simulink model "a3_P1"  (R2023b)
settings: Solver=VariableStepAuto  StartTime=0.0  StopTime=0.2  MaxStep=0.001  RelTol=1e-3
settings Model: Creator=amandeepbehera  LastModifiedBy=amandeepbehera

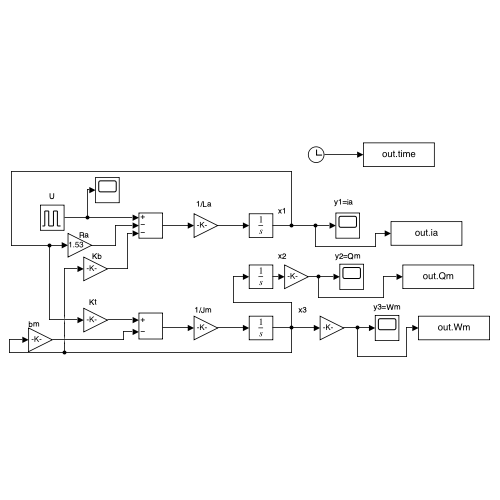
[thumbnail: Simulink's stored preview of the top-level diagram]
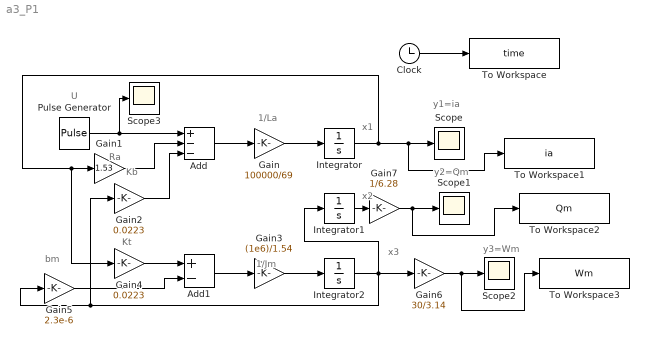
== system a3_P1 ==
  note: y3=Wm
  note: y2=Qm
  note: y1=ia
  note: x3
  note: bm
  note: Kt
  note: 1/Jm
  note: x2
  note: x1
  note: Kb
  note: Ra
  note: U
  note: 1/La
  Add : Sum  Inputs=+--
  Add1 : Sum  Inputs=+-
  Clock : Clock
  Gain : Gain  Gain=100000/69
  Gain1 : Gain  Gain=1.53
  Gain2 : Gain  Gain=0.0223
  Gain3 : Gain  Gain=(1e6)/1.54
  Gain4 : Gain  Gain=0.0223
  Gain5 : Gain  Gain=2.3e-6
  Gain6 : Gain  Gain=30/3.14
  Gain7 : Gain  Gain=1/6.28
  Integrator : Integrator
  Integrator1 : Integrator
  Integrator2 : Integrator
  Pulse Generator : DiscretePulseGenerator  PulseType=Time based  Amplitude=10  Period=.2  PulseWidth=50
  Scope{,1..3} (4 alike) : Scope
  To Workspace : ToWorkspace  VariableName=time  SampleTime=-1
  To Workspace1 : ToWorkspace  VariableName=ia  SampleTime=-1
  To Workspace2 : ToWorkspace  VariableName=Qm  SampleTime=-1
  To Workspace3 : ToWorkspace  VariableName=Wm  SampleTime=-1
  wires:
  Add/1 -> Gain/1
  Gain/1 -> Integrator/1
  Integrator/1 -> To Workspace1/1, Scope/1, Gain4/1, Gain1/1
  Integrator2/1 -> Gain6/1, Integrator1/1, Gain5/1, Gain2/1
  Gain1/1 -> Add/2
  Gain2/1 -> Add/3
  Gain3/1 -> Integrator2/1
  Add1/1 -> Gain3/1
  Gain4/1 -> Add1/1
  Gain5/1 -> Add1/2
  Gain6/1 -> To Workspace3/1, Scope2/1
  Pulse Generator/1 -> Scope3/1, Add/1
  Clock/1 -> To Workspace/1
  Integrator1/1 -> Gain7/1
  Gain7/1 -> To Workspace2/1, Scope1/1
